simulink model "control"  (R2022b)
settings: Solver=VariableStepAuto  StartTime=0.0  StopTime=3.4  RelTol=1e-3
values from neighbouring files (symbols this model uses):
  q0 = [-0.927293431585 -1.28700579042 0.7 2.21429922201]    [generated_traj.mat]    (also in init_traj.m = [-0.927293431584587;-1.287005790420619;0.700000000000000;2.2)
  Ts = 0.001    [generated_traj.mat]    (also in init_traj.m)
undefined symbols (not defined in the file or in its folder): DiscIntNeverNeededParam
settings Model: Creator=giuseppeloianno  LastModifiedBy=pren_
settings DataIOCC: ReturnWorkspaceOutputs=off

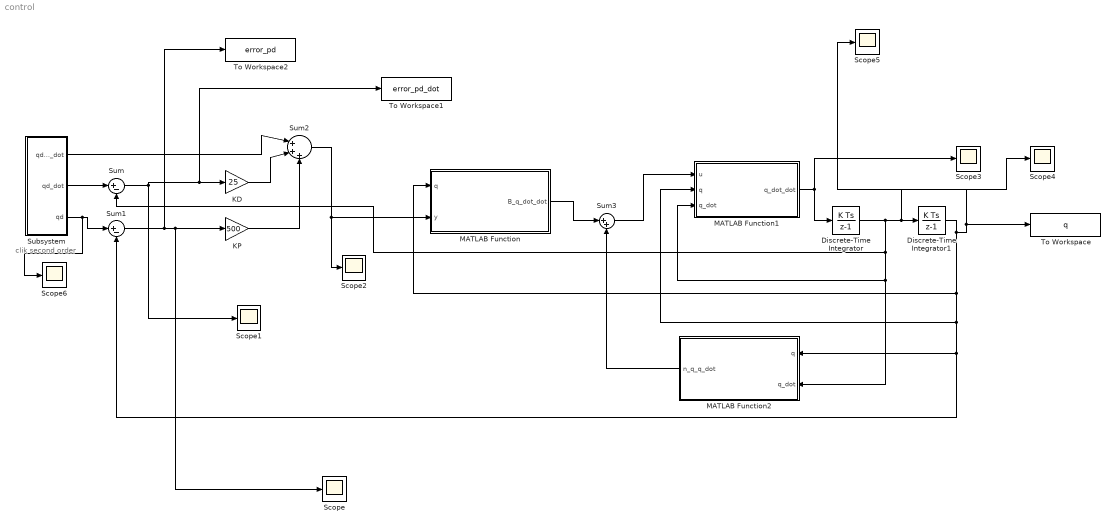
== system control ==
  note: clik second order
  Discrete-Time Integrator : DiscreteIntegrator  InitialCondition=[0;0;0;0]  SampleTime=Ts  ICPrevOutput=DiscIntNeverNeededParam  ICPrevScaledInput=DiscIntNeverNeededParam
  Discrete-Time Integrator1 : DiscreteIntegrator  InitialCondition=q0  SampleTime=Ts  LimitOutput=on  UpperSaturationLimit=[pi/2 *180/pi ;pi/4 *180/pi;1;2*pi *180/pi]  LowerSaturationLimit=[-pi/2 * 180/pi ; -pi/2 * 180/pi ;0.25; -2*pi * 180/pi]  ICPrevOutput=DiscIntNeverNeededParam  ICPrevScaledInput=DiscIntNeverNeededParam
  KD : Gain  Gain=25
  KP : Gain  Gain=500
  MATLAB Function : MATLAB Function  TreatAsAtomicUnit=on
  MATLAB Function1 : MATLAB Function  TreatAsAtomicUnit=on
  MATLAB Function2 : MATLAB Function  TreatAsAtomicUnit=on
  Scope{,1..6} (7 alike) : Scope
  Subsystem : Subsystem
  Sum : Sum  Inputs=|+-
  Sum1 : Sum  Inputs=|+-
  Sum2 : Sum  Inputs=|+++
  Sum3 : Sum  Inputs=|++
  To Workspace : ToWorkspace  VariableName=q  SampleTime=Ts
  To Workspace1 : ToWorkspace  VariableName=error_pd_dot  SampleTime=0.001
  To Workspace2 : ToWorkspace  VariableName=error_pd  SampleTime=0.001
  wires:
  Subsystem/2(qd_dot) -> Sum/1
  Sum/1 -> To Workspace1/1, KD/1, Scope1/1
  Discrete-Time Integrator/1 -> MATLAB Function2/2(q_dot), MATLAB Function1/3(q_dot), Sum/2, Scope4/1, Discrete-Time Integrator1/1
  Subsystem/3(qd) -> Scope6/1, Sum1/1
  Sum1/1 -> Scope/1, KP/1, To Workspace2/1
  Subsystem/1(qd_dot_dot) -> Sum2/1
  KD/1 -> Sum2/2
  KP/1 -> Sum2/3
  Sum2/1 -> Scope2/1, MATLAB Function/2(y)
  MATLAB Function/1(B_q_dot_dot) -> Sum3/1
  Sum3/1 -> MATLAB Function1/1(u)
  MATLAB Function1/1(q_dot_dot) -> Discrete-Time Integrator/1, Scope3/1
  MATLAB Function2/1(n_q_q_dot) -> Sum3/2
  Discrete-Time Integrator1/1 -> Scope5/1, To Workspace/1, MATLAB Function1/2(q), MATLAB Function2/1(q), Sum1/2, MATLAB Function/1(q)

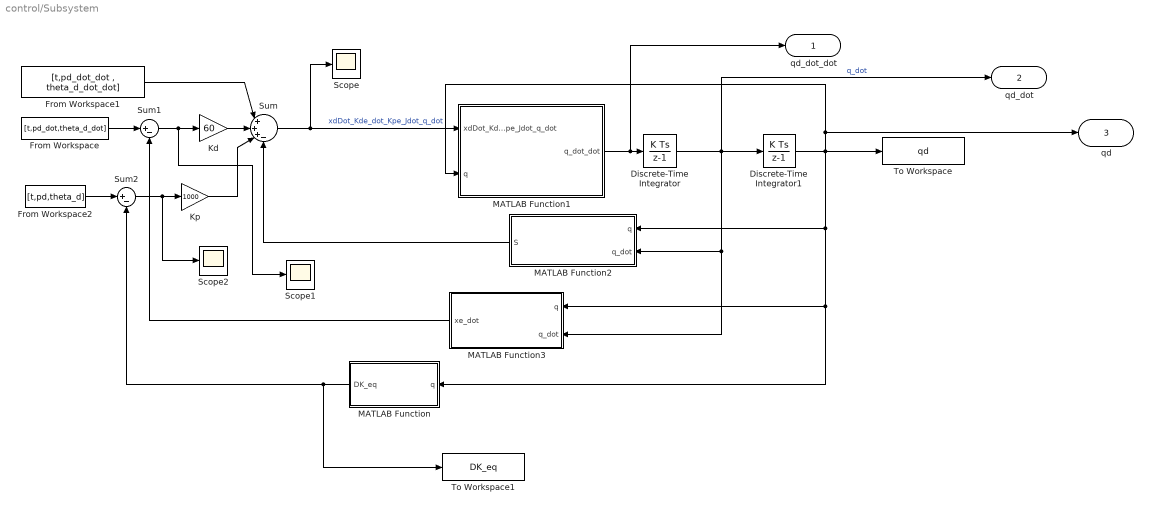
== system control/Subsystem ==
  Discrete-Time Integrator : DiscreteIntegrator  InitialCondition=[0 ;0 ;0; 0]  SampleTime=0.001  UpperSaturationLimit=[pi/2 *180/pi ;pi/4 *180/pi;1;2*pi *180/pi]  LowerSaturationLimit=[-pi/2 * 180/pi ; -pi/2 * 180/pi ;0.25; -2*pi * 180/pi]  ICPrevOutput=DiscIntNeverNeededParam  ICPrevScaledInput=DiscIntNeverNeededParam
  Discrete-Time Integrator1 : DiscreteIntegrator  InitialCondition=q0  SampleTime=Ts  LimitOutput=on  UpperSaturationLimit=[pi/2 *180/pi ;pi/4 *180/pi;1;2*pi *180/pi]  LowerSaturationLimit=[-pi/2 * 180/pi ; -pi/2 * 180/pi ;0.25; -2*pi * 180/pi]  ICPrevOutput=DiscIntNeverNeededParam  ICPrevScaledInput=DiscIntNeverNeededParam
  From Workspace : FromWorkspace  VariableName=[t,pd_dot,theta_d_dot]  OutDataTypeStr=double  SampleTime=0.001
  From Workspace1 : FromWorkspace  VariableName=[t,pd_dot_dot , theta_d_dot_dot]  OutDataTypeStr=double  SampleTime=0.001
  From Workspace2 : FromWorkspace  VariableName=[t,pd,theta_d]  OutDataTypeStr=double  SampleTime=0.001
  Kd : Gain  Gain=60
  Kp : Gain  Gain=1000
  MATLAB Function : MATLAB Function  TreatAsAtomicUnit=on
  MATLAB Function1 : MATLAB Function  TreatAsAtomicUnit=on
  MATLAB Function2 : MATLAB Function  TreatAsAtomicUnit=on
  MATLAB Function3 : MATLAB Function  TreatAsAtomicUnit=on
  Scope : Scope
  Scope1 : Scope
  Scope2 : Scope
  Sum : Sum  Inputs=|+++-
  Sum1 : Sum  Inputs=|+-
  Sum2 : Sum  Inputs=|+-
  To Workspace : ToWorkspace  VariableName=qd  SampleTime=0.001
  To Workspace1 : ToWorkspace  VariableName=DK_eq  SampleTime=-1
  qd_dot_dot : Outport
  qd_dot : Outport  Port=2
  qd : Outport  Port=3
  wires:
  Discrete-Time Integrator1/1 -> MATLAB Function1/2(q), qd/1, MATLAB Function2/1(q), MATLAB Function3/1(q), MATLAB Function/1(q), To Workspace/1
  From Workspace1/1 -> Sum/1
  Kp/1 -> Sum/3
  Discrete-Time Integrator/1 -> qd_dot/1, MATLAB Function2/2(q_dot), MATLAB Function3/2(q_dot), Discrete-Time Integrator1/1  "q_dot"
  Kd/1 -> Sum/2
  From Workspace/1 -> Sum1/1
  Sum/1 -> Scope/1, MATLAB Function1/1(xdDot_Kde_dot_Kpe_Jdot_q_dot)  "xdDot_Kde_dot_Kpe_Jdot_q_dot"
  MATLAB Function/1(DK_eq) -> To Workspace1/1, Sum2/2
  MATLAB Function1/1(q_dot_dot) -> qd_dot_dot/1, Discrete-Time Integrator/1
  MATLAB Function2/1(S) -> Sum/4
  MATLAB Function3/1(xe_dot) -> Sum1/2
  From Workspace2/1 -> Sum2/1
  Sum2/1 -> Scope2/1, Kp/1
  Sum1/1 -> Scope1/1, Kd/1

== matlab function control/Subsystem/MATLAB Function1 ==
  data: xdDot_Kde_dot_Kpe_Jdot_q_dot input; q_dot_dot output; q input
function q_dot_dot  = jacobian_inverse(xdDot_Kde_dot_Kpe_Jdot_q_dot, q)
    q_dot_dot = [0; 0; 0; 0]; %Since q_dot will give 4 outputs (theta1dot , theta2dot, d3dot , theta4dot)
    q_dot_dot= jacobian_inverse(xdDot_Kde_dot_Kpe_Jdot_q_dot ,q);
end

== matlab function control/Subsystem/MATLAB Function ==
  data: q input; DK_eq output
function DK_eq = direct_kin(q)
%coder.extrinsic("direct_kin")
DK_eq= [0 0 0 0];
DK_eq = direct_kin(q);
end

== matlab function control/Subsystem/MATLAB Function2 ==
  data: q input; S output; q_dot input
function S = jacobian_dot(q,q_dot)
    %S = [0 0 0 0];
    S = jacobian_dot(q,q_dot);
end

== matlab function control/Subsystem/MATLAB Function3 ==
  data: q input; q_dot input; xe_dot output
function xe_dot = jacobian(q,q_dot) 
   %[IndJ]= [0 0 0 0 ;0 0 0 0 ; 0 0 0 0 ;0 0 0 0];
   [xe_dot] = [0 ,0, 0, 0];
   [~, xe_dot] = jacobian(q,q_dot);
end

== matlab function control/MATLAB Function ==
  data: q input; y input; B_q_dot_dot output
function B_q_dot_dot = B(q,y)
    B_q_dot_dot = B(q,y);
end

== matlab function control/MATLAB Function1 ==
  data: u input; q_dot_dot output; q input; q_dot input
function q_dot_dot  = manipulator(u,q,q_dot)
    q_dot_dot = manipulator(u,q,q_dot);
end

== matlab function control/MATLAB Function2 ==
  data: q input; q_dot input; n_q_q_dot output
function n_q_q_dot= n(q,q_dot)
    n_q_q_dot= n(q,q_dot);
end
